simulink model "IndustrialMicrogrid"  (R2025a)
settings: Solver=FixedStepAuto  StartTime=0.0  StopTime=8  FixedStep=Ts  RelTol=1e-3
PostLoadFcn:
  | IndustrialMicrogridInputData
  | GfmGridFormingConverterInputParameters
model workspace (MAT data in the model file):
  caseNum = 2
undefined symbols (not defined in the file): base, BESS, DiscIntNeverNeededParam, grid, Grid, gridInverter, machine, microgrid, PV, PVInverter, PVTransformer, scrFactorRg, scrFactorXg, transformer, Transition_and_Dispatch_ControlModeType, Ts
libraries: ee_lib x126, fl_lib x91, eeGeneralControl x73, nesl_utility x50, nesl_utility_internal x46, simulink x30, eeTransforms x11, eeSinusoidalMeasurementV2 x5, eeTotalHarmonicDistorsion x4, slpidlib x3, simulink_extras x2, eePowerMeasurement x2
(part 9 of 12)

== system IndustrialMicrogrid/MG1 Primary Substation/BESS and Controller/BESS/Grid-Forming Converter Control/Power Control ==
  note: Reactive Power Control
  note: Active Power Control
  In Bus Element2 : Inport  PortName=measure  Element=P
  In Bus Element1 : Inport  PortName=measure  Element=fgrid
  BusElementIn : Inport  PortName=measure  Element=Vgd
  BusElementIn2 : Inport  PortName=measure  Element=Q
  Pref : Inport  Port=2
  Qref : Inport  Port=3
  Vref : Inport  Port=4
  Fref : Inport  Port=5
  CntrlFlag : Inport  Port=6
  ActivePowerControl : Subsystem  Variant=on  VariantControlMode=label  VariantControl=Choice  LabelModeActiveChoice=vsm
  ReactiveControl : Subsystem
  Scope : Scope
      settings: ActiveDisplayYMinimum=-0.5584  ActiveDisplayYMaximum=2.30161  DataLoggingVariableName=ScopeData16
  Out Bus Element : Outport  PortName=reactiveControl  Element=Vmd
  Out Bus Element1 : Outport  PortName=reactiveControl  Element=Vmq
  Out Bus Element6 : Outport  Port=2  PortName=activeControl  Element=angle
  Out Bus Element4 : Outport  Port=2  PortName=activeControl  Element=w
  angle : Outport  Port=3
  wires:
  ActivePowerControl/2(w) -> Out Bus Element4/1
  ActivePowerControl/1(Theta) -> angle/1, Out Bus Element6/1
  ReactiveControl/1(Vmd) -> Out Bus Element/1
  ReactiveControl/2(Vmq) -> Out Bus Element1/1
  Pref/1 -> ActivePowerControl/1(Pref)  "Q"
  Qref/1 -> ReactiveControl/2(Qref)  "Q"
  In Bus Element2/1 -> ActivePowerControl/2(Pmeas)
  In Bus Element1/1 -> ActivePowerControl/5(fgrid)
  Fref/1 -> ActivePowerControl/3(fref)
  CntrlFlag/1 -> [Cntrlflag]
  [Cntrlflag] -> ActivePowerControl/4(cntrlflag)
  Vref/1 -> ReactiveControl/5(Vref)
  [Cntrlflag] -> ReactiveControl/1(CntrlFlag)
  BusElementIn/1 -> Scope/1, ReactiveControl/4(Vgdmeas)
  BusElementIn2/1 -> ReactiveControl/3(Qmeas)

== system IndustrialMicrogrid/MG1 Primary Substation/BESS and Controller/BESS/Grid-Forming Converter Control/VoltageCurrentControl ==
  In Bus Element : Inport  PortName=currentLimiting  Element=Vmd
  In Bus Element1 : Inport  PortName=currentLimiting  Element=Vmq
  In Bus Element6 : Inport  PortName=currentLimiting  Element=Idmax
  In Bus Element7 : Inport  PortName=currentLimiting  Element=Iqmax
  Bus Element In6 : Inport  Port=2  PortName=activeControl  Element=w
  Bus Element In1 : Inport  Port=2  PortName=activeControl  Element=angle
  BlackStart : Inport  Port=3
  In Bus Element2 : Inport  Port=4  PortName=measure  Element=Vgd
  In Bus Element3 : Inport  Port=4  PortName=measure  Element=Vgq
  In Bus Element4 : Inport  Port=4  PortName=measure  Element=Igd
  In Bus Element5 : Inport  Port=4  PortName=measure  Element=Igq
  Controller : Subsystem
      settings: PortSchema="{\"entries\":[{\"content\":{\"sides\":[{\"content\":{\"connectorIds\":[\"In1\",\"In2\",\"In3\",\"In4\",\"In5\",\"In6\",\"In7\",\"In8\",\"In9\"]},\"type\":\"ConnectorPlacement.EquallySpacedRectSide\",\"uuid\":\"29d30ab3-0ae0-4ae6-aaee-46c6f5faca9c\"},{\"content\":{\"connectorIds\":[\"Out1\",\"Out2\"],\"side\":\"RIGHT\"},\"type\":\"ConnectorPlacement.EquallySpacedRectSide\",\"uuid\":\"4918c3a7-9f8f-4af5-ac25-a0a0710917b2\"},{\"content\":{\"connectorIds\":[\"In10\"],\"side\":\"TOP\"},\"type\":\"ConnectorPlacement.EquallySpacedRectSide\",\"uuid\":\"c6ee8000-0a39-46c2-b8e8-8b73a56a82d9\"}]},\"type\":\"ConnectorPlacement.EquallySpacedConnector\",\"uuid\":\"193e0bc8-3764-41d1-9278-3938c4a9e9f5\"}],\"packageUris\":[\"http://schema.mathworks.com/mf0/Connector/R2020b\"],\"version\":\"1.0\"}"
  Modulation Signal : Subsystem
  mabc : Outport
  wires:
  Controller/2(Vq) -> Modulation Signal/2(Vq)
  Modulation Signal/1(mabc) -> mabc/1
  Controller/1(Vd) -> Modulation Signal/1(Vd)
  In Bus Element4/1 -> Controller/6(Id)
  In Bus Element5/1 -> Controller/7(Iq)
  In Bus Element6/1 -> Controller/8(Idmax)
  In Bus Element7/1 -> Controller/9(Iqmax)
  In Bus Element2/1 -> Controller/4(Vsd)
  In Bus Element3/1 -> Controller/5(Vsq)
  Bus Element In6/1 -> Controller/1(Angfreq)
  In Bus Element/1 -> Controller/2(Vgdref)
  In Bus Element1/1 -> Controller/3(Vgqref)
  Bus Element In1/1 -> Modulation Signal/3(Angle)
  BlackStart/1 -> Controller/10(BlackStart1)

== system IndustrialMicrogrid/MG2 PV Plant/(500KWp PV)/PV Inverter A2/PV & Inverter/Measurement1 ==
  u : Inport
  Lead-Lag (Discrete or Continuous) : eeGeneralControl/Lead-Lag (Discrete or Continuous)  T1=0  T2=PV.controllerTSensor  B=inf  A=-inf  init_option=Inherited from block input  x0=0  Ts=Ts
      settings: LibrarySourceBlock=|
      | ee_sl_lib/General Control/Lead-Lag
      | (Discrete or Continuous)
  Out1 : Outport
  wires:
  u/1 -> Lead-Lag (Discrete or Continuous)/1
  Lead-Lag (Discrete or Continuous)/1 -> Out1/1

== system IndustrialMicrogrid/MG2 PV Plant/(500KWp PV)/PV Inverter A2/PV & Inverter/Measurement2 ==
  u : Inport
  Lead-Lag (Discrete or Continuous) : eeGeneralControl/Lead-Lag (Discrete or Continuous)  T1=0  T2=PV.controllerTSensor  B=inf  A=-inf  init_option=Inherited from block input  x0=0  Ts=Ts
      settings: LibrarySourceBlock=|
      | ee_sl_lib/General Control/Lead-Lag
      | (Discrete or Continuous)
  Out1 : Outport
  wires:
  u/1 -> Lead-Lag (Discrete or Continuous)/1
  Lead-Lag (Discrete or Continuous)/1 -> Out1/1

== system IndustrialMicrogrid/MG2 PV Plant/(500KWp PV)/PV Inverter A2/PV & Inverter/P&O MPP ==
  In1 : Inport
  Input : Inport  Port=2
  AND1 : Logic  IconShape=distinctive  AllPortsSameDT=off  OutDataTypeStr=boolean
  Add : Sum
  Compare To Zero1 : simulink/Logic and Bit Operations/Compare To Zero  relop=>=  OutDataTypeStr=boolean
  Compare To Zero2 : simulink/Logic and Bit Operations/Compare To Zero  relop=>=  OutDataTypeStr=boolean
  Constant1 : Constant  Value=PV.mppDv
  NOR : Logic  Operator=NOR  IconShape=distinctive  AllPortsSameDT=off  OutDataTypeStr=boolean
  OR : Logic  Operator=OR  IconShape=distinctive  AllPortsSameDT=off  OutDataTypeStr=boolean
  Subtract5 : Sum  Inputs=-+
  Sum : Sum  Inputs=|+-
  Sum1 : Sum  Inputs=|-+
  Switch4 : Switch  Criteria=u2 ~= 0  SaturateOnIntegerOverflow=off  InputSameDT=off
  Switch5 : Switch  Criteria=u2 > Threshold  SaturateOnIntegerOverflow=off  InputSameDT=off
  Unit Delay : UnitDelay  InitialCondition=2.5e5  SampleTime=PV.mppTs  HasFrameUpgradeWarning=on
  Unit Delay1 : UnitDelay  InitialCondition=1*PVInverter.Vdc  SampleTime=PV.mppTs  HasFrameUpgradeWarning=on
  ZOH/3 : ZeroOrderHold  SampleTime=0.02
  start MPPT Voltage : Constant  Value=PVInverter.Vdc  SampleTime=Ts
  Vmpp : Outport  VectorParamsAs1DForOutWhenUnconnected=off
  wires:
  [Vinc] -> Switch4/1
  ZOH/3/1 -> Vmpp/1
  Unit Delay/1 -> Sum/2
  AND1/1 -> OR/1
  Sum/1 -> Compare To Zero2/1
  Sum1/1 -> Compare To Zero1/1
  Switch4/1 -> ZOH/3/1
  [Vdec] -> Switch4/3
  Subtract5/1 -> [Vdec]  "DEC"
  NOR/1 -> OR/2
  Add/1 -> [Vinc]  "INC"
  Unit Delay1/1 -> Sum1/1
  Input/1 -> Unit Delay1/1, Sum1/2, Switch5/1, Switch5/2
  Constant1/1 -> Subtract5/1, Add/2
  Switch5/1 -> Subtract5/2, Add/1
  In1/1 -> Sum/1, Unit Delay/1
  Compare To Zero2/1 -> AND1/1, NOR/2
  start MPPT Voltage/1 -> Switch5/3
  Compare To Zero1/1 -> AND1/2, NOR/1
  OR/1 -> Switch4/2

== system IndustrialMicrogrid/MG2 PV Plant/(500KWp PV)/PV Inverter A2/PV Controller/Current_controller ==
  id-ref : Inport
  ipvd : Inport  Port=2
  iqref : Inport  Port=3
  iq : Inport  Port=4
  Vd : Inport  Port=5
  Vq : Inport  Port=6
  Constant4 : Constant  Value=0
  Gain1 : Gain  Gain=2*1*pi*60*PVInverter.l/PV.zBase
  Gain2 : Gain  Gain=2*1*pi*60*PVInverter.l/PV.zBase
  Mux1 : Mux  Inputs=3
  PID Controller : slpidlib/PID Controller  Controller=PID  Form=Parallel  TimeDomain=Discrete-time  UseExternalTs=off  SampleTime=-1  IntegratorMethod=Forward Euler  FilterMethod=Forward Euler  ControllerParametersSource=internal  P=PV.controllerKpIc*0.02*2  I=PV.controllerKiIc*0.02*2  UseKiTs=off  D=PV.controllerKd  UseExternalDerivativeSource=off  N=100  UseFilter=off  TunerSelectOption=Transfer Function Based (PID Tuner App)  InitialConditionSource=internal  InitialConditionForIntegrator=-0.023  InitialConditionForFilter=0  DifferentiatorICPrevScaledInput=0  ExternalReset=none  TrackingMode=off  Kt=1  LimitOutput=off  SatLimitsSource=internal  UpperSaturationLimit=1.5  LowerSaturationLimit=-1.5  LinearizeAsGain=on  AntiWindupMode=clamping  Kb=1  LimitIntegrator=off  UpperIntegratorSaturationLimit=1.5  LowerIntegratorSaturationLimit=-1.5  POutMin=[]  POutMax=[]  IOutMin=[]  IOutMax=[]  DOutMin=[]  DOutMax=[]  NOutMin=[]  NOutMax=[]  SumOutMin=[]  SumOutMax=[]  SaturationOutMin=[]  SaturationOutMax=[]  PParamMin=[]  PParamMax=[]  IParamMin=[]  IParamMax=[]  DParamMin=[]  DParamMax=[]  NParamMin=[]  NParamMax=[]  KbParamMin=[]  KbParamMax=[]  KtParamMin=[]  KtParamMax=[]  KbOutMin=[]  KbOutMax=[]  KtOutMin=[]  KtOutMax=[]  IntegratorOutMin=[]  IntegratorOutMax=[]  FilterOutMin=[]  FilterOutMax=[]  SumI1OutMin=[]  SumI1OutMax=[]  SumI2OutMin=[]  SumI2OutMax=[]  SumI3OutMin=[]  SumI3OutMax=[]  SumI4OutMin=[]  SumI4OutMax=[]  SumDOutMin=[]  SumDOutMax=[]  DifferentiatorOutMin=[]  DifferentiatorOutMax=[]  FilterDiffOutCoefMin=[]  FilterDiffOutCoefMax=[]  ReciprocalOutMin=[]  ReciprocalOutMax=[]  SumDenOutMin=[]  SumDenOutMax=[]  SumNumOutMin=[]  SumNumOutMax=[]  DivideOutMin=[]  DivideOutMax=[]  UdiffTsProdOutMin=[]  UdiffTsProdOutMax=[]  NTsProdOutMin=[]  NTsProdOutMax=[]  UintegralTsProdOutMin=[]  UintegralTsProdOutMax=[]  UngainTsProdOutMin=[]  UngainTsProdOutMax=[]  ClampingZeroOutDataTypeStr=Inherit: Inherit via back propagation  ClampingZeroOutMin=[]  ClampingZeroOutMax=[]  FilterDenConstantOutDataTypeStr=Inherit: Inherit via back propagation  FilterDenConstantOutMin=[]  FilterDenConstantOutMax=[]  PCopyOutDataTypeStr=Inherit: Inherit via back propagation  PCopyOutMin=[]  PCopyOutMax=[]  NCopyOutDataTypeStr=Inherit: Inherit via back propagation  NCopyOutMin=[]  NCopyOutMax=[]  IntegratorContinuousStateAttributes=''  IntegratorStateMustResolveToSignalObject=off  IntegratorRTWStateStorageClass=Auto  FilterContinuousStateAttributes=''  FilterStateMustResolveToSignalObject=off  FilterRTWStateStorageClass=Auto  ParallelPVariant=InternalParameters  IdealPVariant=Disabled  IVariant=InternalParameters  DVariant=InternalParameters  IntegratorVariant=Discrete  SatVariant=Disabled  AWVariant=Passthrough  PCopyVariant=Disabled  TRVariant=Disabled  FdbkBlocksVariant=Forward  IdealPFdbkVariant=Disabled  SatFdbkVariant=Disabled  DerivativeFilterVariant=Differentiator  NVariant=Passthrough  NCopyVariant=Disabled_SignalSpec  FilterICVariant=InternalICsDifferentiator  IntegratorICVariant=InternalICs  ExternalResetVariant=Disabled  TRSumVariant=Passthrough  SumFdbkVariant=Disabled  SumVariant=Sum_PID  TsampFilterVariant=InternalTs  TsampNgainVariant=Passthrough  TsampIntegralVariant=Disabled_SignalSpec  ExternalSaturationOutDataTypeStr=Inherit: Same as second input  DerivativeSourceVariant=ErrorSignal  PreIntVariant=InternalPreInt
  PID Controller1 : slpidlib/PID Controller  Controller=PID  Form=Parallel  TimeDomain=Discrete-time  UseExternalTs=off  SampleTime=-1  IntegratorMethod=Forward Euler  FilterMethod=Forward Euler  ControllerParametersSource=internal  P=PV.controllerKpIc*10  I=PV.controllerKiIc*0.2  UseKiTs=off  D=PV.controllerKd  UseExternalDerivativeSource=off  N=100  UseFilter=off  TunerSelectOption=Transfer Function Based (PID Tuner App)  InitialConditionSource=internal  InitialConditionForIntegrator=0.4  InitialConditionForFilter=0  DifferentiatorICPrevScaledInput=0  ExternalReset=none  TrackingMode=off  Kt=1  LimitOutput=off  SatLimitsSource=internal  UpperSaturationLimit=1.5  LowerSaturationLimit=-1.5  LinearizeAsGain=on  AntiWindupMode=clamping  Kb=1  LimitIntegrator=off  UpperIntegratorSaturationLimit=1.5  LowerIntegratorSaturationLimit=-1.5  POutMin=[]  POutMax=[]  IOutMin=[]  IOutMax=[]  DOutMin=[]  DOutMax=[]  NOutMin=[]  NOutMax=[]  SumOutMin=[]  SumOutMax=[]  SaturationOutMin=[]  SaturationOutMax=[]  PParamMin=[]  PParamMax=[]  IParamMin=[]  IParamMax=[]  DParamMin=[]  DParamMax=[]  NParamMin=[]  NParamMax=[]  KbParamMin=[]  KbParamMax=[]  KtParamMin=[]  KtParamMax=[]  KbOutMin=[]  KbOutMax=[]  KtOutMin=[]  KtOutMax=[]  IntegratorOutMin=[]  IntegratorOutMax=[]  FilterOutMin=[]  FilterOutMax=[]  SumI1OutMin=[]  SumI1OutMax=[]  SumI2OutMin=[]  SumI2OutMax=[]  SumI3OutMin=[]  SumI3OutMax=[]  SumI4OutMin=[]  SumI4OutMax=[]  SumDOutMin=[]  SumDOutMax=[]  DifferentiatorOutMin=[]  DifferentiatorOutMax=[]  FilterDiffOutCoefMin=[]  FilterDiffOutCoefMax=[]  ReciprocalOutMin=[]  ReciprocalOutMax=[]  SumDenOutMin=[]  SumDenOutMax=[]  SumNumOutMin=[]  SumNumOutMax=[]  DivideOutMin=[]  DivideOutMax=[]  UdiffTsProdOutMin=[]  UdiffTsProdOutMax=[]  NTsProdOutMin=[]  NTsProdOutMax=[]  UintegralTsProdOutMin=[]  UintegralTsProdOutMax=[]  UngainTsProdOutMin=[]  UngainTsProdOutMax=[]  ClampingZeroOutDataTypeStr=Inherit: Inherit via back propagation  ClampingZeroOutMin=[]  ClampingZeroOutMax=[]  FilterDenConstantOutDataTypeStr=Inherit: Inherit via back propagation  FilterDenConstantOutMin=[]  FilterDenConstantOutMax=[]  PCopyOutDataTypeStr=Inherit: Inherit via back propagation  PCopyOutMin=[]  PCopyOutMax=[]  NCopyOutDataTypeStr=Inherit: Inherit via back propagation  NCopyOutMin=[]  NCopyOutMax=[]  IntegratorContinuousStateAttributes=''  IntegratorStateMustResolveToSignalObject=off  IntegratorRTWStateStorageClass=Auto  FilterContinuousStateAttributes=''  FilterStateMustResolveToSignalObject=off  FilterRTWStateStorageClass=Auto  ParallelPVariant=InternalParameters  IdealPVariant=Disabled  IVariant=InternalParameters  DVariant=InternalParameters  IntegratorVariant=Discrete  SatVariant=Disabled  AWVariant=Passthrough  PCopyVariant=Disabled  TRVariant=Disabled  FdbkBlocksVariant=Forward  IdealPFdbkVariant=Disabled  SatFdbkVariant=Disabled  DerivativeFilterVariant=Differentiator  NVariant=Passthrough  NCopyVariant=Disabled_SignalSpec  FilterICVariant=InternalICsDifferentiator  IntegratorICVariant=InternalICs  ExternalResetVariant=Disabled  TRSumVariant=Passthrough  SumFdbkVariant=Disabled  SumVariant=Sum_PID  TsampFilterVariant=InternalTs  TsampNgainVariant=Passthrough  TsampIntegralVariant=Disabled_SignalSpec  ExternalSaturationOutDataTypeStr=Inherit: Same as second input  DerivativeSourceVariant=ErrorSignal  PreIntVariant=InternalPreInt
  Sum1 : Sum  Inputs=|+-
  Sum3 : Sum  Inputs=|++-
  Sum4 : Sum  Inputs=|+++
  Sum5 : Sum  Inputs=|+-
  Refrence_mdq0 : Outport
  wires:
  ipvd/1 -> Sum1/2, Gain1/1
  id-ref/1 -> Sum1/1
  iq/1 -> Sum5/2, Gain2/1
  iqref/1 -> Sum5/1
  Vd/1 -> Sum3/1
  Vq/1 -> Sum4/2
  Mux1/1 -> Refrence_mdq0/1  "m_dqo"
  Sum4/1 -> Mux1/2
  PID Controller1/1 -> Sum4/1
  Sum5/1 -> PID Controller1/1
  Constant4/1 -> Mux1/3
  Sum1/1 -> PID Controller/1
  Gain1/1 -> Sum4/3
  Gain2/1 -> Sum3/3
  Sum3/1 -> Mux1/1
  PID Controller/1 -> Sum3/2

== system IndustrialMicrogrid/MG2 PV Plant/(500KWp PV)/PV Inverter A2/PV Controller/DC voltage controller & current reference ==
  note: id_ref_generator
  note: iq_ref_generator
  note: Limiter
  Q_ref : Inport
  Vmag : Inport  Port=2
  P_pv : Inport  Port=3
  PV_Mpp_vdc : Inport  Port=4
  PV_vdc : Inport  Port=5
  LVRT.iq : Inport  Port=6
  Constant : Constant
  Constant1 : Constant  Value=PVInverter.iMaxPU
  Current limits : Subsystem
  Subsystem : Subsystem
  Subsystem1 : Subsystem
  Switch : Switch  Criteria=u2 > Threshold  SaturateOnIntegerOverflow=off  InputSameDT=off
  Unit Delay1 : UnitDelay  SampleTime=Ts  HasFrameUpgradeWarning=on
  Unit Delay3 : UnitDelay  SampleTime=Ts  HasFrameUpgradeWarning=on
  iq_ref : Outport
  id_ref : Outport  Port=2
  wires:
  Constant/1 -> Switch/3
  Switch/1 -> Subsystem1/1(Vmag), Subsystem/1(V_mag)
  Vmag/1 -> Switch/1, Switch/2
  LVRT.iq/1 -> Subsystem/3(LVRT.iq)
  [ubiq] -> Subsystem/2(iq_ub)
  [ubid] -> Subsystem1/5(id_ub)
  Subsystem/1(Out1) -> iq_ref/1, [iq_ref]
  PV_vdc/1 -> Subsystem1/4(PV_vdc)
  PV_Mpp_vdc/1 -> Subsystem1/3(PV_Mpp_vdc)
  P_pv/1 -> Subsystem1/2(P_pv)
  Subsystem1/1(Out1) -> id_ref/1, [id_ref]
  Q_ref/1 -> Subsystem/4(Q_ref)
  Unit Delay3/1 -> Current limits/3(idref)
  [id_ref] -> Unit Delay3/1
  Unit Delay1/1 -> Current limits/2(iqref)
  Constant1/1 -> Current limits/1(Imax)
  Current limits/1(iubd) -> [ubid]
  Current limits/2(iubq) -> [ubiq]
  [iq_ref] -> Unit Delay1/1

== system IndustrialMicrogrid/MG2 Primary Substation/BESS and Controller/BESS/Grid-Forming Converter Control/Current Limiting ==
  In Bus Element : Inport  PortName=measure  Element=Igd
  In Bus Element1 : Inport  PortName=measure  Element=Igq
  In Bus Element2 : Inport  Port=2  PortName=reactiveControl  Element=Vmd
  In Bus Element4 : Inport  Port=2  PortName=reactiveControl  Element=Vmq
  CurrentLimitingMethod : Subsystem  Variant=on  VariantControlMode=label  VariantControl=Choice  LabelModeActiveChoice=virimp
  Subtract : Sum  Inputs=+-
  Subtract1 : Sum  Inputs=-+
  Out Bus Element : Outport  PortName=currentLimiting  Element=Vmd
  Out Bus Element1 : Outport  PortName=currentLimiting  Element=Vmq
  Out Bus Element2 : Outport  PortName=currentLimiting  Element=Idmax
  Out Bus Element3 : Outport  PortName=currentLimiting  Element=Iqmax
  wires:
  In Bus Element2/1 -> Subtract/1
  In Bus Element1/1 -> CurrentLimitingMethod/2(Igq)
  In Bus Element4/1 -> Subtract1/2
  Subtract/1 -> Out Bus Element/1
  Subtract1/1 -> Out Bus Element1/1
  CurrentLimitingMethod/4(Iqmax) -> Out Bus Element3/1
  In Bus Element/1 -> CurrentLimitingMethod/1(Igd)  "Q"
  CurrentLimitingMethod/3(Idmax) -> Out Bus Element2/1
  CurrentLimitingMethod/1(delVd) -> Subtract/2
  CurrentLimitingMethod/2(delVq) -> Subtract1/1

== system IndustrialMicrogrid/MG2 Primary Substation/BESS and Controller/BESS/Grid-Forming Converter Control/Grid Voltage Reactive Power Support ==
  In Bus Element1 : Inport  PortName=measure  Element=Vgd
  In Bus Element3 : Inport  PortName=measure  Element=Vgq
  In Bus Element2 : Inport  PortName=measure  Element=Igd
  In Bus Element4 : Inport  PortName=measure  Element=Igq
  PrefInput : Inport  Port=2
  QrefInput : Inport  Port=3
  Modifying Active Power Reference : Subsystem
  Modifying Reactive Power Reference : Subsystem
  Pref : Outport
  Qref : Outport  Port=2
  wires:
  Modifying Active Power Reference/1(Pref) -> Modifying Reactive Power Reference/4(Pref)
  PrefInput/1 -> Modifying Active Power Reference/1(PrefInput)
  In Bus Element2/1 -> Modifying Active Power Reference/3(Igd)
  In Bus Element4/1 -> Modifying Active Power Reference/4(Igq)
  In Bus Element1/1 -> Modifying Reactive Power Reference/1(Vgd), Modifying Active Power Reference/2(Vd)
  In Bus Element3/1 -> Modifying Reactive Power Reference/2(Vgq)
  QrefInput/1 -> Modifying Reactive Power Reference/3(Qref)
  Modifying Reactive Power Reference/1(PrefNew) -> Pref/1
  Modifying Reactive Power Reference/2(QrefNew) -> Qref/1

== system IndustrialMicrogrid/MG2 Primary Substation/BESS and Controller/BESS/Grid-Forming Converter Control/Measurement ==
  Vgabcc : Inport
  Igabc : Inport  Port=2
  Angle : Inport  Port=3
  Frequency Measurement : Subsystem
  Gain1 : Gain  Gain=1/power
  Gain2 : Gain  Gain=1/power
  Gain3 : Gain  Gain=1/(girdLineVoltage*sqrt(2/3))
  Gain4 : Gain  Gain=1/(girdLineVoltage*sqrt(2/3))
  Gain5 : Gain  Gain=1/(power/(sqrt(3)*girdLineVoltage)*sqrt(2))
  Gain6 : Gain  Gain=1/(power/(sqrt(3)*girdLineVoltage)*sqrt(2))
  Power Measurement (Three-Phase) : eePowerMeasurement/Power Measurement (Three-Phase)  LabelModeActiveChoice=Discrete  F=powerFreq  K=[1]  Seq=Positive  Ts=measSampleTime
  abc2dq : Subsystem
  Out Bus Element : Outport  PortName=measure  Element=P
  Out Bus Element1 : Outport  PortName=measure  Element=Q
  Out Bus Element2 : Outport  PortName=measure  Element=Vgd
  Out Bus Element3 : Outport  PortName=measure  Element=Vgq
  Out Bus Element4 : Outport  PortName=measure  Element=Igd
  Out Bus Element5 : Outport  PortName=measure  Element=Igq
  Out Bus Element6 : Outport  PortName=measure  Element=fgrid
  Pmeas : Outport  Port=2
  Qmeas : Outport  Port=3
  fmeas : Outport  Port=4
  wires:
  Vgabcc/1 -> abc2dq/3(Vgabc), Frequency Measurement/1(Vabc), Power Measurement (Three-Phase)/1  "Vabc"
  Angle/1 -> abc2dq/2(Angle)
  Power Measurement (Three-Phase)/1 -> Gain2/1
  Igabc/1 -> abc2dq/1(Igabc), Power Measurement (Three-Phase)/2  "Iabc"
  Power Measurement (Three-Phase)/2 -> Gain1/1
  Gain2/1 -> Pmeas/1, Out Bus Element/1  "Pmeas"
  Gain1/1 -> Qmeas/1, Out Bus Element1/1  "Qmeas"
  abc2dq/1(Vgd) -> Gain4/1
  abc2dq/2(Vgq) -> Gain3/1
  abc2dq/3(Igd) -> Gain5/1
  abc2dq/4(Igq) -> Gain6/1
  Gain3/1 -> Out Bus Element3/1  "Vgq"
  Gain4/1 -> Out Bus Element2/1  "Vgd"
  Gain5/1 -> Out Bus Element4/1  "Igd"
  Gain6/1 -> Out Bus Element5/1  "Igq"
  Frequency Measurement/1(freq) -> Out Bus Element6/1, fmeas/1

== system IndustrialMicrogrid/MG2 Primary Substation/BESS and Controller/BESS/Grid-Forming Converter Control/Power Control ==
  note: Reactive Power Control
  note: Active Power Control
  In Bus Element2 : Inport  PortName=measure  Element=P
  In Bus Element1 : Inport  PortName=measure  Element=fgrid
  BusElementIn : Inport  PortName=measure  Element=Vgd
  BusElementIn2 : Inport  PortName=measure  Element=Q
  Pref : Inport  Port=2
  Qref : Inport  Port=3
  Vref : Inport  Port=4
  Fref : Inport  Port=5
  CntrlFlag : Inport  Port=6
  ActivePowerControl : Subsystem  Variant=on  VariantControlMode=label  VariantControl=Choice  LabelModeActiveChoice=vsm
  ReactiveControl : Subsystem
  Scope : Scope
      settings: ActiveDisplayYMinimum=-13.20558  ActiveDisplayYMaximum=19.03908  DataLoggingVariableName=ScopeData16
  Out Bus Element : Outport  PortName=reactiveControl  Element=Vmd
  Out Bus Element1 : Outport  PortName=reactiveControl  Element=Vmq
  Out Bus Element6 : Outport  Port=2  PortName=activeControl  Element=angle
  Out Bus Element4 : Outport  Port=2  PortName=activeControl  Element=w
  angle : Outport  Port=3
  wires:
  ActivePowerControl/2(w) -> Out Bus Element4/1
  ActivePowerControl/1(Theta) -> angle/1, Out Bus Element6/1
  ReactiveControl/1(Vmd) -> Out Bus Element/1
  ReactiveControl/2(Vmq) -> Out Bus Element1/1
  Pref/1 -> ActivePowerControl/1(Pref)  "Q"
  Qref/1 -> ReactiveControl/2(Qref)  "Q"
  In Bus Element2/1 -> ActivePowerControl/2(Pmeas)
  In Bus Element1/1 -> ActivePowerControl/5(fgrid)
  Fref/1 -> ActivePowerControl/3(fref)
  CntrlFlag/1 -> [Cntrlflag]
  [Cntrlflag] -> ActivePowerControl/4(cntrlflag)
  Vref/1 -> ReactiveControl/5(Vref)
  [Cntrlflag] -> ReactiveControl/1(CntrlFlag)
  BusElementIn/1 -> Scope/1, ReactiveControl/4(Vgdmeas)
  BusElementIn2/1 -> ReactiveControl/3(Qmeas)

== system IndustrialMicrogrid/MG2 Primary Substation/BESS and Controller/BESS/Grid-Forming Converter Control/VoltageCurrentControl ==
  In Bus Element : Inport  PortName=currentLimiting  Element=Vmd
  In Bus Element1 : Inport  PortName=currentLimiting  Element=Vmq
  In Bus Element6 : Inport  PortName=currentLimiting  Element=Idmax
  In Bus Element7 : Inport  PortName=currentLimiting  Element=Iqmax
  Bus Element In6 : Inport  Port=2  PortName=activeControl  Element=w
  Bus Element In1 : Inport  Port=2  PortName=activeControl  Element=angle
  BlackStart : Inport  Port=3
  In Bus Element2 : Inport  Port=4  PortName=measure  Element=Vgd
  In Bus Element3 : Inport  Port=4  PortName=measure  Element=Vgq
  In Bus Element4 : Inport  Port=4  PortName=measure  Element=Igd
  In Bus Element5 : Inport  Port=4  PortName=measure  Element=Igq
  Controller : Subsystem
      settings: PortSchema="{\"entries\":[{\"content\":{\"sides\":[{\"content\":{\"connectorIds\":[\"In1\",\"In2\",\"In3\",\"In4\",\"In5\",\"In6\",\"In7\",\"In8\",\"In9\"]},\"type\":\"ConnectorPlacement.EquallySpacedRectSide\",\"uuid\":\"29d30ab3-0ae0-4ae6-aaee-46c6f5faca9c\"},{\"content\":{\"connectorIds\":[\"Out1\",\"Out2\"],\"side\":\"RIGHT\"},\"type\":\"ConnectorPlacement.EquallySpacedRectSide\",\"uuid\":\"4918c3a7-9f8f-4af5-ac25-a0a0710917b2\"},{\"content\":{\"connectorIds\":[\"In10\"],\"side\":\"TOP\"},\"type\":\"ConnectorPlacement.EquallySpacedRectSide\",\"uuid\":\"c6ee8000-0a39-46c2-b8e8-8b73a56a82d9\"}]},\"type\":\"ConnectorPlacement.EquallySpacedConnector\",\"uuid\":\"193e0bc8-3764-41d1-9278-3938c4a9e9f5\"}],\"packageUris\":[\"http://schema.mathworks.com/mf0/Connector/R2020b\"],\"version\":\"1.0\"}"
  Modulation Signal : Subsystem
  mabc : Outport
  wires:
  Controller/2(Vq) -> Modulation Signal/2(Vq)
  Modulation Signal/1(mabc) -> mabc/1
  Controller/1(Vd) -> Modulation Signal/1(Vd)
  In Bus Element4/1 -> Controller/6(Id)
  In Bus Element5/1 -> Controller/7(Iq)
  In Bus Element6/1 -> Controller/8(Idmax)
  In Bus Element7/1 -> Controller/9(Iqmax)
  In Bus Element2/1 -> Controller/4(Vsd)
  In Bus Element3/1 -> Controller/5(Vsq)
  Bus Element In6/1 -> Controller/1(Angfreq)
  In Bus Element/1 -> Controller/2(Vgdref)
  In Bus Element1/1 -> Controller/3(Vgqref)
  Bus Element In1/1 -> Modulation Signal/3(Angle)
  BlackStart/1 -> Controller/10(BlackStart1)

== system IndustrialMicrogrid/MG1 Primary Substation/BESS and Controller/BESS/Grid-Forming Converter Control/Current Limiting/CurrentLimitingMethod ==
  Igd : Inport
  Igq : Inport  Port=2
  currentLimitAndVirtual : Subsystem  VariantControl=both
  currentSaturation : Subsystem  VariantControl=ctSat
  virtualImpedance : Subsystem  VariantControl=virimp
  delVd : Outport
  delVq : Outport  Port=2
  Idmax : Outport  Port=3
  Iqmax : Outport  Port=4

== system IndustrialMicrogrid/MG1 Primary Substation/BESS and Controller/BESS/Grid-Forming Converter Control/Grid Voltage Reactive Power Support/Modifying Active Power Reference ==
  PrefInput : Inport
  Vd : Inport  Port=2
  Igd : Inport  Port=3
  Igq : Inport  Port=4
  AND : Logic  IconShape=distinctive  AllPortsSameDT=off  OutDataTypeStr=boolean
  Abs : Abs  SaturateOnIntegerOverflow=off
  Compare To Constant : simulink/Logic and Bit Operations/Compare To Constant  relop=>=  const=0.95  OutDataTypeStr=boolean
  Computing New Active Power Ref : Subsystem
  Math Function1 : Math  Operator=hypot
  Power Sign : Signum
  Product : Product
  Relay : Relay  OnSwitchValue=maxVICurrentLimit*0.96  OffSwitchValue=1
  Switch : Switch  Criteria=u2 > Threshold  SaturateOnIntegerOverflow=off  InputSameDT=off
  Pref : Outport
  wires:
  Computing New Active Power Ref/1(Pref) -> Switch/1
  Math Function1/1 -> Relay/1  "Is"
  Vd/1 -> Computing New Active Power Ref/2(Vd), Compare To Constant/1
  PrefInput/1 -> Power Sign/1, Switch/3
  Igd/1 -> Math Function1/2
  Igq/1 -> Computing New Active Power Ref/1(Iq), Math Function1/1
  Switch/1 -> Abs/1
  Abs/1 -> Product/1
  Power Sign/1 -> Product/2
  Product/1 -> Pref/1
  Relay/1 -> AND/2
  AND/1 -> Switch/2
  Compare To Constant/1 -> AND/1

== system IndustrialMicrogrid/MG1 Primary Substation/BESS and Controller/BESS/Grid-Forming Converter Control/Grid Voltage Reactive Power Support/Modifying Reactive Power Reference ==
  Vgd : Inport
  Vgq : Inport  Port=2
  Qref : Inport  Port=3
  Pref : Inport  Port=4
  Changing the Power Reference : Subsystem
  Hysteresis : Subsystem
  Math Function : Math  Operator=hypot
  Merge : Merge
  Merge1 : Merge
  NOT : Logic  Operator=NOT  IconShape=distinctive  AllPortsSameDT=off  OutDataTypeStr=boolean
  Not Altering the Power Reference : Subsystem
  PrefNew : Outport
  QrefNew : Outport  Port=2
  wires:
  Vgd/1 -> [Vd], Math Function/1
  Not Altering the Power Reference/2(Qrefv) -> Merge1/2
  Math Function/1 -> Hysteresis/1(Vs), [Vs]
  [Vs] -> Changing the Power Reference/1(Vs)
  Not Altering the Power Reference/1(Prefv) -> Merge/2
  Changing the Power Reference/1(Prefv) -> Merge/1
  NOT/1 -> Not Altering the Power Reference/Enable
  Qref/1 -> Not Altering the Power Reference/2(Qref), [Qref]
  Hysteresis/1(LVFlag) -> Changing the Power Reference/Enable, NOT/1
  [Vd] -> Changing the Power Reference/2(Vd)
  Changing the Power Reference/2(Qrefv) -> Merge1/1
  Vgq/1 -> Math Function/2
  Pref/1 -> Not Altering the Power Reference/1(Pref), [Pref]
  Merge1/1 -> QrefNew/1
  Merge/1 -> PrefNew/1
  [Pref] -> Changing the Power Reference/3(Pref)
  [Qref] -> Changing the Power Reference/4(Qref)

== system IndustrialMicrogrid/MG1 Primary Substation/BESS and Controller/BESS/Grid-Forming Converter Control/Measurement/Frequency Measurement ==
  Vabc : Inport
  Convert To PU : Gain  Gain=1/powerFreq
  Frequency Measurement : Subsystem  TreatAsAtomicUnit=on  SystemSampleTime=sampleTime  mask{initialFrequency=powerFreq, sampleTime=activePowerSampleTime}
      mask prompts: initialFrequency "Initial frequency in Hz"; sampleTime "Sample time in sec"
      mask DialogControl Container7 Prompt: General
  Low-Pass Filter : eeGeneralControl/Low-Pass Filter (Discrete or Continuous)  K=1  T=freqMeasTimeConst  B=inf  A=-inf  init_option=Inherited from block input  x0=0  Ts=-1
  freq : Outport
  wires:
  Low-Pass Filter/1 -> Convert To PU/1  "Freq"
  Frequency Measurement/1(Freq) -> Low-Pass Filter/1
  Convert To PU/1 -> freq/1
  Vabc/1 -> Frequency Measurement/1(abc)

== system IndustrialMicrogrid/MG1 Primary Substation/BESS and Controller/BESS/Grid-Forming Converter Control/Measurement/abc2dq ==
  Igabc : Inport
  Angle : Inport  Port=2
  Vgabc : Inport  Port=3
  Supply Current to dq : Subsystem
  Supply Voltage  to dq1 : Subsystem
  Vgd : Outport
  Vgq : Outport  Port=2
  Igd : Outport  Port=3
  Igq : Outport  Port=4
  wires:
  Angle/1 -> Supply Voltage  to dq1/1(Angle), Supply Current to dq/2(Angle)
  Vgabc/1 -> Supply Voltage  to dq1/2(abc)
  Igabc/1 -> Supply Current to dq/1(abc)
  Supply Current to dq/1(Igd) -> Igd/1  "Id"
  Supply Current to dq/2(Igq) -> Igq/1  "Iq"
  Supply Voltage  to dq1/1(Vgd) -> Vgd/1  "Vgd"
  Supply Voltage  to dq1/2(Vgq) -> Vgq/1  "Vgq"

== system IndustrialMicrogrid/MG1 Primary Substation/BESS and Controller/BESS/Grid-Forming Converter Control/Power Control/ActivePowerControl ==
  Pref : Inport
  Pmeas : Inport  Port=2
  fref : Inport  Port=3
  cntrlflag : Inport  Port=4
  fgrid : Inport  Port=5
  droopControl : Subsystem  VariantControl=droop
  vsmControl : Subsystem  VariantControl=vsm
  Theta : Outport
  w : Outport  Port=2

== system IndustrialMicrogrid/MG1 Primary Substation/BESS and Controller/BESS/Grid-Forming Converter Control/Power Control/ReactiveControl ==
  note: Vs-delV
  CntrlFlag : Inport
  Qref : Inport  Port=2
  Qmeas : Inport  Port=3
  Vgdmeas : Inport  Port=4
  Vref : Inport  Port=5
  Constant2 : Constant  Value=0
  Saturation1 : Saturate  UpperLimit=(dcBusVoltage/2)/(sqrt(2/3)*girdLineVoltage)  LowerLimit=-(dcBusVoltage/2)/(sqrt(2/3)*girdLineVoltage)
  Scope : Scope
      settings: ActiveDisplayYMinimum=-0.1625  ActiveDisplayYMaximum=1.4625  DataLoggingVariableName=ScopeData20
  Voltage  Reference Selection : Subsystem
  Vmd : Outport
  Vmq : Outport  Port=2
  wires:
  Voltage  Reference Selection/1(Vd) -> Saturation1/1  "Q"
  Constant2/1 -> Vmq/1
  Saturation1/1 -> Scope/1, Vmd/1
  CntrlFlag/1 -> Voltage  Reference Selection/1(cntrlflag)
  Qref/1 -> Voltage  Reference Selection/2(Qref)
  Qmeas/1 -> Voltage  Reference Selection/3(Qmeas)
  Vref/1 -> Voltage  Reference Selection/4(Vref)
  Vgdmeas/1 -> Voltage  Reference Selection/5(Vgdmeas)

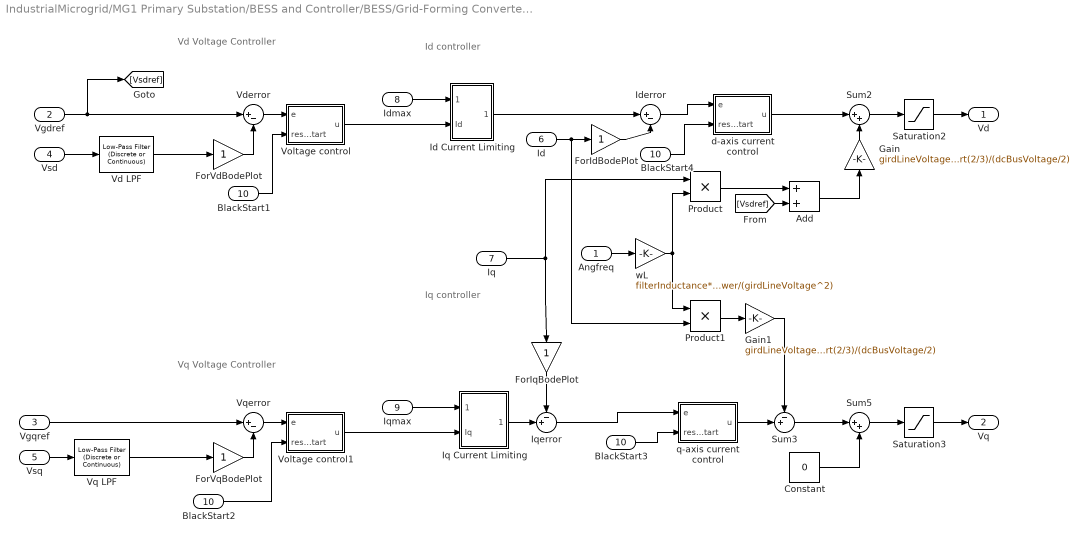
== system IndustrialMicrogrid/MG1 Primary Substation/BESS and Controller/BESS/Grid-Forming Converter Control/VoltageCurrentControl/Controller ==
  note: Id controller
  note: Vd Voltage Controller
  note: Iq controller
  note: Vq Voltage Controller
  Angfreq : Inport
  Vgdref : Inport  Port=2
  Vgqref : Inport  Port=3
  Vsd : Inport  Port=4
  Vsq : Inport  Port=5
  Id : Inport  Port=6
  Iq : Inport  Port=7
  Idmax : Inport  Port=8
  Iqmax : Inport  Port=9
  BlackStart1 : Inport  Port=10
  Add : Sum
  BlackStart2 : InportShadow  Port=10
  BlackStart3 : InportShadow  Port=10
  BlackStart4 : InportShadow  Port=10
  Constant : Constant  Value=0  SampleTime=currentControlTs
  ForIdBodePlot : Gain
  ForIqBodePlot : Gain
  ForVdBodePlot : Gain
  ForVqBodePlot : Gain
  Gain : Gain  Gain=girdLineVoltage*sqrt(2/3)/(dcBusVoltage/2)
  Gain1 : Gain  Gain=girdLineVoltage*sqrt(2/3)/(dcBusVoltage/2)
  Id Current Limiting : Subsystem
  Iderror : Sum  Inputs=|+-
  Iq Current Limiting : Subsystem
  Iqerror : Sum  Inputs=-+|
  Product : Product
  Product1 : Product
  Saturation2 : Saturate  UpperLimit=4  LowerLimit=-3
  Saturation3 : Saturate  UpperLimit=3  LowerLimit=-3
  Sum2 : Sum  Inputs=|++
  Sum3 : Sum  Inputs=-+|
  Sum5 : Sum  Inputs=|++
  Vd LPF : eeGeneralControl/Low-Pass Filter (Discrete or Continuous)  K=1  T=vdvqLPFTimeConst  B=inf  A=-inf  init_option=Specify as parameter  x0=0  Ts=voltControlTs
  Vderror : Sum  Inputs=|+-
  Voltage control : Subsystem
  Voltage control1 : Subsystem
  Vq LPF : eeGeneralControl/Low-Pass Filter (Discrete or Continuous)  K=1  T=vdvqLPFTimeConst  B=inf  A=-inf  init_option=Inherited from block input  x0=0  Ts=voltControlTs
  Vqerror : Sum  Inputs=|+-
  d-axis current control : Subsystem
  q-axis current control : Subsystem
  wL : Gain  Gain=filterInductance*power/(girdLineVoltage^2)
  Vd : Outport  VectorParamsAs1DForOutWhenUnconnected=off
  Vq : Outport  Port=2  VectorParamsAs1DForOutWhenUnconnected=off
  wires:
  Iqerror/1 -> q-axis current control/1(e)
  wL/1 -> Product1/1, Product/2
  Iq/1 -> ForIqBodePlot/1, Product/1
  Angfreq/1 -> wL/1
  Constant/1 -> Sum5/2
  Iderror/1 -> d-axis current control/1(e)
  Saturation3/1 -> Vq/1
  Saturation2/1 -> Vd/1
  Product1/1 -> Gain1/1
  Product/1 -> Add/1
  d-axis current control/1(u) -> Sum2/1
  Sum2/1 -> Saturation2/1
  q-axis current control/1(u) -> Sum3/2
  Sum3/1 -> Sum5/1
  Sum5/1 -> Saturation3/1
  Vsq/1 -> Vq LPF/1
  Id/1 -> Product1/2, ForIdBodePlot/1
  Vderror/1 -> Voltage control/1(e)
  Iqmax/1 -> Iq Current Limiting/1(Imax)
  Vgqref/1 -> Vqerror/1
  Vqerror/1 -> Voltage control1/1(e)
  Gain1/1 -> Sum3/1
  [Vsdref] -> Add/2
  Add/1 -> Gain/1
  Gain/1 -> Sum2/2
  Voltage control/1(u) -> Id Current Limiting/2(Id)
  Idmax/1 -> Id Current Limiting/1(Imax)
  Iq Current Limiting/1(Iqref) -> Iqerror/2
  Voltage control1/1(u) -> Iq Current Limiting/2(Iq)
  Vsd/1 -> Vd LPF/1
  ForVdBodePlot/1 -> Vderror/2
  ForVqBodePlot/1 -> Vqerror/2
  ForIdBodePlot/1 -> Iderror/2
  ForIqBodePlot/1 -> Iqerror/1
  Id Current Limiting/1(Idref) -> Iderror/1
  Vd LPF/1 -> ForVdBodePlot/1
  Vq LPF/1 -> ForVqBodePlot/1
  BlackStart1/1 -> Voltage control/2(resetBlackStart)
  BlackStart2/1 -> Voltage control1/2(resetBlackStart)
  BlackStart3/1 -> q-axis current control/2(resetBlackStart)
  BlackStart4/1 -> d-axis current control/2(resetBlackStart)
  Vgdref/1 -> Vderror/1, [Vsdref]

== system IndustrialMicrogrid/MG1 Primary Substation/BESS and Controller/BESS/Grid-Forming Converter Control/VoltageCurrentControl/Modulation Signal ==
  Vd : Inport
  Vq : Inport  Port=2
  Angle : Inport  Port=3
  Constant : Constant  Value=0
  Inverse Park Transform : eeTransforms/Inverse Park Transform  AxisAlignment=D-axis  PowerInvariant=off
  Mux1 : Mux  Inputs=3
  Saturation2 : Saturate  UpperLimit=1  LowerLimit=-1
  mabc : Outport  VectorParamsAs1DForOutWhenUnconnected=off
  wires:
  Inverse Park Transform/1 -> Saturation2/1
  Mux1/1 -> Inverse Park Transform/1
  Angle/1 -> Inverse Park Transform/2
  Saturation2/1 -> mabc/1
  Constant/1 -> Mux1/3
  Vd/1 -> Mux1/1
  Vq/1 -> Mux1/2

== system IndustrialMicrogrid/MG2 PV Plant/(500KWp PV)/PV Inverter A2/PV Controller/DC voltage controller & current reference/Current limits ==
  Imax : Inport
  iqref : Inport  Port=2
  idref : Inport  Port=3
  Constant8 : Constant  Value=0
  Constant9 : Constant  Value=0
  Sqrt : Sqrt
  Sqrt1 : Sqrt
  Square{1..4} (4 alike) : Math  Operator=square
  Step2 : Step  Time=0.01  SampleTime=Ts
  Step3 : Step  Time=0.01  SampleTime=Ts
  Sum6 : Sum  Inputs=|+-
  Sum9 : Sum  Inputs=|+-
  Switch1 : Switch  Threshold=.01  SaturateOnIntegerOverflow=off  InputSameDT=off
  Switch2 : Switch  Threshold=.01  SaturateOnIntegerOverflow=off  InputSameDT=off
  iubd : Outport
  iubq : Outport  Port=2
  wires:
  idref/1 -> Square4/1
  Sqrt1/1 -> iubq/1
  Imax/1 -> Square1/1, Square3/1
  Sqrt/1 -> iubd/1
  Constant9/1 -> Switch2/3
  Square4/1 -> Sum9/2
  Constant8/1 -> Switch1/3
  Square2/1 -> Sum6/2
  Sum6/1 -> Switch1/1
  Square3/1 -> Sum9/1
  iqref/1 -> Square2/1
  Switch1/1 -> Sqrt/1
  Square1/1 -> Sum6/1
  Switch2/1 -> Sqrt1/1
  Step2/1 -> Switch1/2
  Step3/1 -> Switch2/2
  Sum9/1 -> Switch2/1

== system IndustrialMicrogrid/MG2 PV Plant/(500KWp PV)/PV Inverter A2/PV Controller/DC voltage controller & current reference/Subsystem ==
  V_mag : Inport
  iq_ub : Inport  Port=2
  LVRT.iq : Inport  Port=3
  Q_ref : Inport  Port=4
  Divide2 : Product  Inputs=*/
  Gain3 : Gain  Gain=-1
  Low-Pass Filter (Discrete or Continuous)1 : eeGeneralControl/Low-Pass Filter (Discrete or Continuous)  K=1  T=0.04  B=inf  A=-inf  init_option=Inherited from block input  x0=0  Ts=-1
  Saturation Dynamic2 : simulink/Discontinuities/Saturation Dynamic  OutMin=[]  OutMax=[]  OutDataTypeStr=Inherit: Same as second input  OutDataType=fixdt(1, 16)  OutScaling=2^-10  DoSatur=off
  Switch6 : Switch  Threshold=.9  SaturateOnIntegerOverflow=off  InputSameDT=off
  iq_ub1 : InportShadow  Port=2
  Out1 : Outport
  wires:
  Low-Pass Filter (Discrete or Continuous)1/1 -> Divide2/2, Switch6/2
  LVRT.iq/1 -> Switch6/3
  Switch6/1 -> Out1/1
  Saturation Dynamic2/1 -> Switch6/1
  iq_ub/1 -> Saturation Dynamic2/1
  Gain3/1 -> Saturation Dynamic2/3
  Q_ref/1 -> Divide2/1
  Divide2/1 -> Saturation Dynamic2/2
  iq_ub1/1 -> Gain3/1
  V_mag/1 -> Low-Pass Filter (Discrete or Continuous)1/1

== system IndustrialMicrogrid/MG2 PV Plant/(500KWp PV)/PV Inverter A2/PV Controller/DC voltage controller & current reference/Subsystem1 ==
  Vmag : Inport
  P_pv : Inport  Port=2
  PV_Mpp_vdc : Inport  Port=3
  PV_vdc : Inport  Port=4
  id_ub : Inport  Port=5
  Constant4 : Constant  Value=0
  Divide : Product  Inputs=/*
  Gain4 : Gain  Gain=1/(PV.MVABaseNew)
  Low-Pass Filter (Discrete or Continuous) : eeGeneralControl/Low-Pass Filter (Discrete or Continuous)  K=1  T=0.1  B=inf  A=-inf  init_option=Inherited from block input  x0=0  Ts=-1
  Low-Pass Filter (Discrete or Continuous)1 : eeGeneralControl/Low-Pass Filter (Discrete or Continuous)  K=1  T=0.1  B=inf  A=-inf  init_option=Inherited from block input  x0=0  Ts=-1
  Low-Pass Filter (Discrete or Continuous)2 : eeGeneralControl/Low-Pass Filter (Discrete or Continuous)  K=1  T=0.2  B=inf  A=-inf  init_option=Inherited from block input  x0=0  Ts=-1
  Low-Pass Filter (Discrete or Continuous)3 : eeGeneralControl/Low-Pass Filter (Discrete or Continuous)  K=1  T=0.2  B=inf  A=-inf  init_option=Inherited from block input  x0=0  Ts=-1
  Saturation Dynamic1 : simulink/Discontinuities/Saturation Dynamic  OutMin=[]  OutMax=[]  OutDataTypeStr=Inherit: Same as second input  OutDataType=fixdt(1, 16)  OutScaling=2^-10  DoSatur=off
  Sum : Sum  Inputs=|++
  V_dc_Controller1 : Subsystem
  Out1 : Outport
  wires:
  Low-Pass Filter (Discrete or Continuous)3/1 -> V_dc_Controller1/1(PV_plant1)
  Low-Pass Filter (Discrete or Continuous)2/1 -> V_dc_Controller1/2(In2)
  Low-Pass Filter (Discrete or Continuous)1/1 -> Divide/1
  Low-Pass Filter (Discrete or Continuous)/1 -> Gain4/1
  PV_Mpp_vdc/1 -> Low-Pass Filter (Discrete or Continuous)3/1
  Saturation Dynamic1/1 -> Out1/1
  Divide/1 -> Sum/1
  Gain4/1 -> Divide/2
  id_ub/1 -> Saturation Dynamic1/1
  PV_vdc/1 -> Low-Pass Filter (Discrete or Continuous)2/1
  Vmag/1 -> Low-Pass Filter (Discrete or Continuous)1/1
  Sum/1 -> Saturation Dynamic1/2
  V_dc_Controller1/1(Out1) -> Sum/2
  P_pv/1 -> Low-Pass Filter (Discrete or Continuous)/1
  Constant4/1 -> Saturation Dynamic1/3

== system IndustrialMicrogrid/MG2 Primary Substation/BESS and Controller/BESS/Grid-Forming Converter Control/Current Limiting/CurrentLimitingMethod ==
  Igd : Inport
  Igq : Inport  Port=2
  currentLimitAndVirtual : Subsystem  VariantControl=both
  currentSaturation : Subsystem  VariantControl=ctSat
  virtualImpedance : Subsystem  VariantControl=virimp
  delVd : Outport
  delVq : Outport  Port=2
  Idmax : Outport  Port=3
  Iqmax : Outport  Port=4

== system IndustrialMicrogrid/MG2 Primary Substation/BESS and Controller/BESS/Grid-Forming Converter Control/Grid Voltage Reactive Power Support/Modifying Active Power Reference ==
  PrefInput : Inport
  Vd : Inport  Port=2
  Igd : Inport  Port=3
  Igq : Inport  Port=4
  AND : Logic  IconShape=distinctive  AllPortsSameDT=off  OutDataTypeStr=boolean
  Abs : Abs  SaturateOnIntegerOverflow=off
  Compare To Constant : simulink/Logic and Bit Operations/Compare To Constant  relop=>=  const=0.95  OutDataTypeStr=boolean
  Computing New Active Power Ref : Subsystem
  Math Function1 : Math  Operator=hypot
  Power Sign : Signum
  Product : Product
  Relay : Relay  OnSwitchValue=maxVICurrentLimit*0.96  OffSwitchValue=1
  Switch : Switch  Criteria=u2 > Threshold  SaturateOnIntegerOverflow=off  InputSameDT=off
  Pref : Outport
  wires:
  Computing New Active Power Ref/1(Pref) -> Switch/1
  Math Function1/1 -> Relay/1  "Is"
  Vd/1 -> Computing New Active Power Ref/2(Vd), Compare To Constant/1
  PrefInput/1 -> Power Sign/1, Switch/3
  Igd/1 -> Math Function1/2
  Igq/1 -> Computing New Active Power Ref/1(Iq), Math Function1/1
  Switch/1 -> Abs/1
  Abs/1 -> Product/1
  Power Sign/1 -> Product/2
  Product/1 -> Pref/1
  Relay/1 -> AND/2
  AND/1 -> Switch/2
  Compare To Constant/1 -> AND/1

== system IndustrialMicrogrid/MG2 Primary Substation/BESS and Controller/BESS/Grid-Forming Converter Control/Grid Voltage Reactive Power Support/Modifying Reactive Power Reference ==
  Vgd : Inport
  Vgq : Inport  Port=2
  Qref : Inport  Port=3
  Pref : Inport  Port=4
  Changing the Power Reference : Subsystem
  Hysteresis : Subsystem
  Math Function : Math  Operator=hypot
  Merge : Merge
  Merge1 : Merge
  NOT : Logic  Operator=NOT  IconShape=distinctive  AllPortsSameDT=off  OutDataTypeStr=boolean
  Not Altering the Power Reference : Subsystem
  PrefNew : Outport
  QrefNew : Outport  Port=2
  wires:
  Vgd/1 -> [Vd], Math Function/1
  Not Altering the Power Reference/2(Qrefv) -> Merge1/2
  Math Function/1 -> Hysteresis/1(Vs), [Vs]
  [Vs] -> Changing the Power Reference/1(Vs)
  Not Altering the Power Reference/1(Prefv) -> Merge/2
  Changing the Power Reference/1(Prefv) -> Merge/1
  NOT/1 -> Not Altering the Power Reference/Enable
  Qref/1 -> Not Altering the Power Reference/2(Qref), [Qref]
  Hysteresis/1(LVFlag) -> Changing the Power Reference/Enable, NOT/1
  [Vd] -> Changing the Power Reference/2(Vd)
  Changing the Power Reference/2(Qrefv) -> Merge1/1
  Vgq/1 -> Math Function/2
  Pref/1 -> Not Altering the Power Reference/1(Pref), [Pref]
  Merge1/1 -> QrefNew/1
  Merge/1 -> PrefNew/1
  [Pref] -> Changing the Power Reference/3(Pref)
  [Qref] -> Changing the Power Reference/4(Qref)

== system IndustrialMicrogrid/MG2 Primary Substation/BESS and Controller/BESS/Grid-Forming Converter Control/Measurement/Frequency Measurement ==
  Vabc : Inport
  Convert To PU : Gain  Gain=1/powerFreq
  Frequency Measurement : Subsystem  TreatAsAtomicUnit=on  SystemSampleTime=sampleTime  mask{initialFrequency=powerFreq, sampleTime=activePowerSampleTime}
      mask prompts: initialFrequency "Initial frequency in Hz"; sampleTime "Sample time in sec"
      mask DialogControl Container7 Prompt: General
  Low-Pass Filter : eeGeneralControl/Low-Pass Filter (Discrete or Continuous)  K=1  T=freqMeasTimeConst  B=inf  A=-inf  init_option=Inherited from block input  x0=0  Ts=-1
  freq : Outport
  wires:
  Low-Pass Filter/1 -> Convert To PU/1  "Freq"
  Frequency Measurement/1(Freq) -> Low-Pass Filter/1
  Convert To PU/1 -> freq/1
  Vabc/1 -> Frequency Measurement/1(abc)

== system IndustrialMicrogrid/MG2 Primary Substation/BESS and Controller/BESS/Grid-Forming Converter Control/Measurement/abc2dq ==
  Igabc : Inport
  Angle : Inport  Port=2
  Vgabc : Inport  Port=3
  Supply Current to dq : Subsystem
  Supply Voltage  to dq1 : Subsystem
  Vgd : Outport
  Vgq : Outport  Port=2
  Igd : Outport  Port=3
  Igq : Outport  Port=4
  wires:
  Angle/1 -> Supply Voltage  to dq1/1(Angle), Supply Current to dq/2(Angle)
  Vgabc/1 -> Supply Voltage  to dq1/2(abc)
  Igabc/1 -> Supply Current to dq/1(abc)
  Supply Current to dq/1(Igd) -> Igd/1  "Id"
  Supply Current to dq/2(Igq) -> Igq/1  "Iq"
  Supply Voltage  to dq1/1(Vgd) -> Vgd/1  "Vgd"
  Supply Voltage  to dq1/2(Vgq) -> Vgq/1  "Vgq"

== system IndustrialMicrogrid/MG2 Primary Substation/BESS and Controller/BESS/Grid-Forming Converter Control/Power Control/ActivePowerControl ==
  Pref : Inport
  Pmeas : Inport  Port=2
  fref : Inport  Port=3
  cntrlflag : Inport  Port=4
  fgrid : Inport  Port=5
  droopControl : Subsystem  VariantControl=droop
  vsmControl : Subsystem  VariantControl=vsm
  Theta : Outport
  w : Outport  Port=2

== system IndustrialMicrogrid/MG2 Primary Substation/BESS and Controller/BESS/Grid-Forming Converter Control/Power Control/ReactiveControl ==
  note: Vs-delV
  CntrlFlag : Inport
  Qref : Inport  Port=2
  Qmeas : Inport  Port=3
  Vgdmeas : Inport  Port=4
  Vref : Inport  Port=5
  Constant2 : Constant  Value=0
  Saturation1 : Saturate  UpperLimit=(dcBusVoltage/2)/(sqrt(2/3)*girdLineVoltage)  LowerLimit=-(dcBusVoltage/2)/(sqrt(2/3)*girdLineVoltage)
  Scope : Scope
      settings: ActiveDisplayYMinimum=-0.1625  ActiveDisplayYMaximum=1.4625  DataLoggingVariableName=ScopeData20
  Voltage  Reference Selection : Subsystem
  Vmd : Outport
  Vmq : Outport  Port=2
  wires:
  Voltage  Reference Selection/1(Vd) -> Saturation1/1  "Q"
  Constant2/1 -> Vmq/1
  Saturation1/1 -> Scope/1, Vmd/1
  CntrlFlag/1 -> Voltage  Reference Selection/1(cntrlflag)
  Qref/1 -> Voltage  Reference Selection/2(Qref)
  Qmeas/1 -> Voltage  Reference Selection/3(Qmeas)
  Vref/1 -> Voltage  Reference Selection/4(Vref)
  Vgdmeas/1 -> Voltage  Reference Selection/5(Vgdmeas)

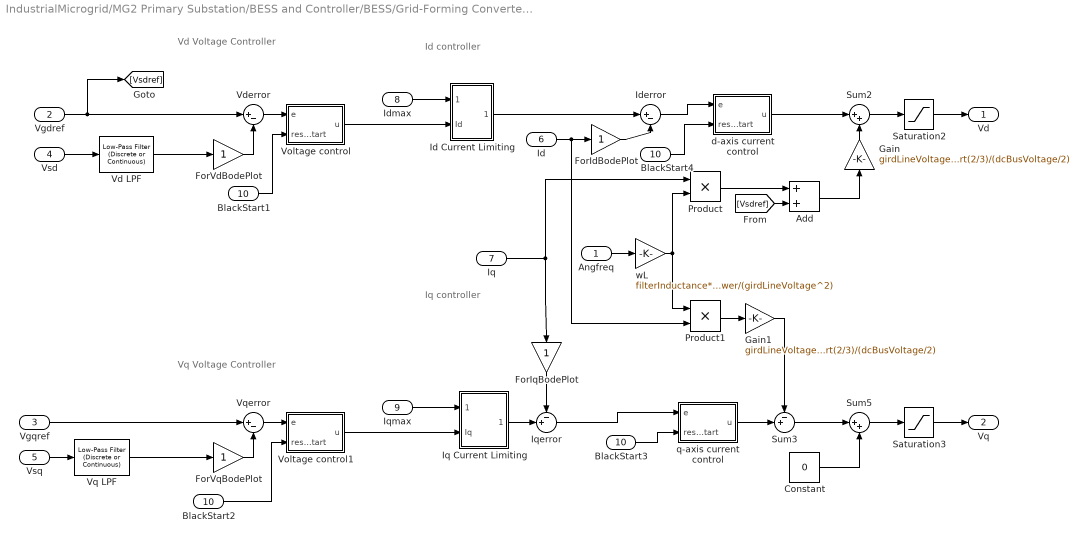
== system IndustrialMicrogrid/MG2 Primary Substation/BESS and Controller/BESS/Grid-Forming Converter Control/VoltageCurrentControl/Controller ==
  note: Id controller
  note: Vd Voltage Controller
  note: Iq controller
  note: Vq Voltage Controller
  Angfreq : Inport
  Vgdref : Inport  Port=2
  Vgqref : Inport  Port=3
  Vsd : Inport  Port=4
  Vsq : Inport  Port=5
  Id : Inport  Port=6
  Iq : Inport  Port=7
  Idmax : Inport  Port=8
  Iqmax : Inport  Port=9
  BlackStart1 : Inport  Port=10
  Add : Sum
  BlackStart2 : InportShadow  Port=10
  BlackStart3 : InportShadow  Port=10
  BlackStart4 : InportShadow  Port=10
  Constant : Constant  Value=0  SampleTime=currentControlTs
  ForIdBodePlot : Gain
  ForIqBodePlot : Gain
  ForVdBodePlot : Gain
  ForVqBodePlot : Gain
  Gain : Gain  Gain=girdLineVoltage*sqrt(2/3)/(dcBusVoltage/2)
  Gain1 : Gain  Gain=girdLineVoltage*sqrt(2/3)/(dcBusVoltage/2)
  Id Current Limiting : Subsystem
  Iderror : Sum  Inputs=|+-
  Iq Current Limiting : Subsystem
  Iqerror : Sum  Inputs=-+|
  Product : Product
  Product1 : Product
  Saturation2 : Saturate  UpperLimit=4  LowerLimit=-3
  Saturation3 : Saturate  UpperLimit=3  LowerLimit=-3
  Sum2 : Sum  Inputs=|++
  Sum3 : Sum  Inputs=-+|
  Sum5 : Sum  Inputs=|++
  Vd LPF : eeGeneralControl/Low-Pass Filter (Discrete or Continuous)  K=1  T=vdvqLPFTimeConst  B=inf  A=-inf  init_option=Specify as parameter  x0=0  Ts=voltControlTs
  Vderror : Sum  Inputs=|+-
  Voltage control : Subsystem
  Voltage control1 : Subsystem
  Vq LPF : eeGeneralControl/Low-Pass Filter (Discrete or Continuous)  K=1  T=vdvqLPFTimeConst  B=inf  A=-inf  init_option=Inherited from block input  x0=0  Ts=voltControlTs
  Vqerror : Sum  Inputs=|+-
  d-axis current control : Subsystem
  q-axis current control : Subsystem
  wL : Gain  Gain=filterInductance*power/(girdLineVoltage^2)
  Vd : Outport  VectorParamsAs1DForOutWhenUnconnected=off
  Vq : Outport  Port=2  VectorParamsAs1DForOutWhenUnconnected=off
  wires:
  Iqerror/1 -> q-axis current control/1(e)
  wL/1 -> Product1/1, Product/2
  Iq/1 -> ForIqBodePlot/1, Product/1
  Angfreq/1 -> wL/1
  Constant/1 -> Sum5/2
  Iderror/1 -> d-axis current control/1(e)
  Saturation3/1 -> Vq/1
  Saturation2/1 -> Vd/1
  Product1/1 -> Gain1/1
  Product/1 -> Add/1
  d-axis current control/1(u) -> Sum2/1
  Sum2/1 -> Saturation2/1
  q-axis current control/1(u) -> Sum3/2
  Sum3/1 -> Sum5/1
  Sum5/1 -> Saturation3/1
  Vsq/1 -> Vq LPF/1
  Id/1 -> Product1/2, ForIdBodePlot/1
  Vderror/1 -> Voltage control/1(e)
  Iqmax/1 -> Iq Current Limiting/1(Imax)
  Vgqref/1 -> Vqerror/1
  Vqerror/1 -> Voltage control1/1(e)
  Gain1/1 -> Sum3/1
  [Vsdref] -> Add/2
  Add/1 -> Gain/1
  Gain/1 -> Sum2/2
  Voltage control/1(u) -> Id Current Limiting/2(Id)
  Idmax/1 -> Id Current Limiting/1(Imax)
  Iq Current Limiting/1(Iqref) -> Iqerror/2
  Voltage control1/1(u) -> Iq Current Limiting/2(Iq)
  Vsd/1 -> Vd LPF/1
  ForVdBodePlot/1 -> Vderror/2
  ForVqBodePlot/1 -> Vqerror/2
  ForIdBodePlot/1 -> Iderror/2
  ForIqBodePlot/1 -> Iqerror/1
  Id Current Limiting/1(Idref) -> Iderror/1
  Vd LPF/1 -> ForVdBodePlot/1
  Vq LPF/1 -> ForVqBodePlot/1
  BlackStart1/1 -> Voltage control/2(resetBlackStart)
  BlackStart2/1 -> Voltage control1/2(resetBlackStart)
  BlackStart3/1 -> q-axis current control/2(resetBlackStart)
  BlackStart4/1 -> d-axis current control/2(resetBlackStart)
  Vgdref/1 -> Vderror/1, [Vsdref]
